simulink library "Tools"  (Simulink 8.0)
settings: Solver=ode45  StartTime=0.0  StopTime=10.0  RelTol=1e-3
libraries: simulink x1
settings Model: Creator=h3now  LastModifiedBy=h3now

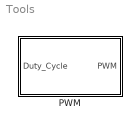
== system Tools ==
  PWM : Subsystem  StartFcn=|  mask{f=20000}
      | T_PWM = get_param(gcb,'f');                                             
      | T_PWM = 1./str2double(T_PWM);                                           
      | T_solver = get_param(bdroot,'FixedStep');                               
      | T_solver = str2double(T_solver);                                        
      | if T_solver > 0.5*T_PWM                                                 
      |    %error('Solver step size must be smaller than 10% of the PWM period')
      | end
      mask prompts: f "PWM Frequency [Hz}"
      mask help:
      | Simula o funcionamento de um PWM.
      |
      | Duty_Cycle = Sinal que varia entre 0 e 1 e define o duty cycle do PWM.

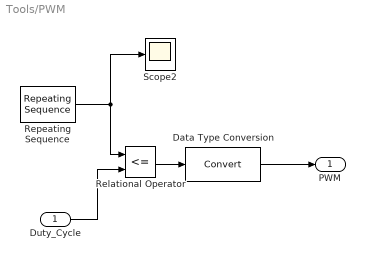
== system Tools/PWM ==
  Duty_Cycle : Inport
  Data Type Conversion : DataTypeConversion
  Relational Operator : RelationalOperator  Operator=<=  OutDataTypeStr=boolean
  Repeating Sequence : simulink/Sources/Repeating Sequence  rep_seq_t=[0 1/f]  rep_seq_y=[0 1]
  Scope2 : Scope
      settings: YMin=0.294  YMax=0.301
  PWM : Outport
  wires:
  Relational Operator/1 -> Data Type Conversion/1
  Data Type Conversion/1 -> PWM/1
  Repeating Sequence/1 -> Relational Operator/1, Scope2/1
  Duty_Cycle/1 -> Relational Operator/2
